simulink model "fu_simu_png_radome_origin"  (R2020a)
settings: Solver=ode4  StartTime=0.0  StopTime=20  FixedStep=0.001  RelTol=1e-3
values from neighbouring files (symbols this model uses):
  N = 4    [initial.m]
  T_alpha = 1    [initial.m]
  tau = 0.1    [initial.m]
  V_M = 500    [initial.m]
libraries: simulink x1
settings Model: Creator=admin  LastModifiedBy=anwaei

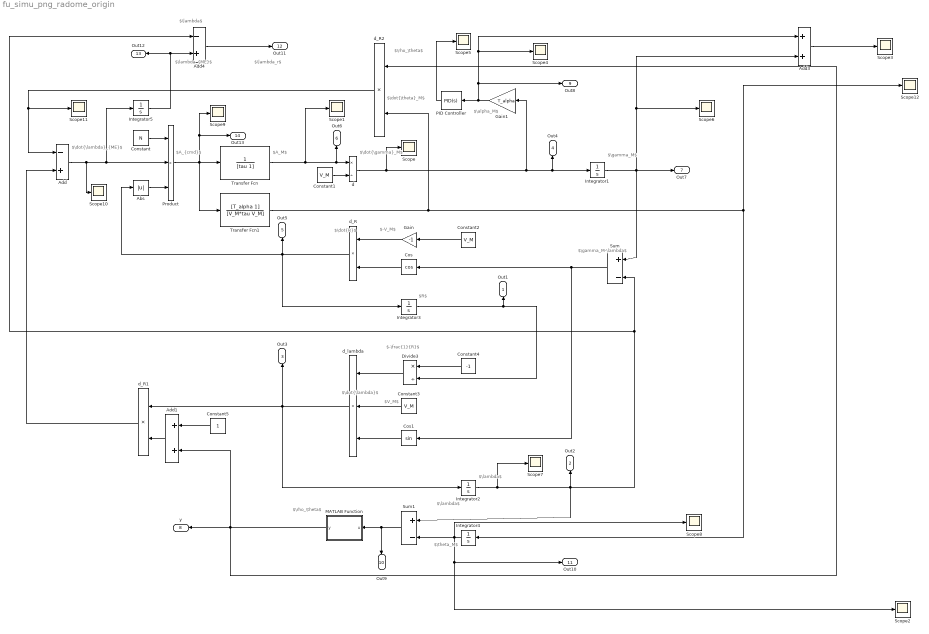
== system fu_simu_png_radome_origin ==
  note: $\dot{\lambda}$
  note: $\lambda$
  note: $\gamma_M$
  note: $-\frac{1}{R}$
  note: $V_M$
  note: $\gamma_M-\lambda$
  note: $-V_M$
  note: $\dot{R}$
  note: $A_{cmd}$
  note: $A_M$
  note: $\dot{\gamma}_M$
  note: $R$
  note: $\dot{\theta}_M$
  note: $\dot{\lambda}_{ME}$
  note: $\theta_M$
  note: $\lambda$
  note: $\rho_\theta$
  note: $\rho_\theta$
  note: $\alpha_M$
  note: $\lambda_{ME}$
  note: $\lambda$
  note: $\lambda_r$
  Abs : Abs
  Add : Sum  Inputs=-+
  Add1 : Sum
  Add3 : Sum
  Add4 : Sum  Inputs=-+
  Constant : Constant  Value=N
  Constant1 : Constant  Value=V_M
  Constant2 : Constant  Value=V_M
  Constant3 : Constant  Value=V_M
  Constant4 : Constant  Value=-1
  Constant5 : Constant
  Cos : Trigonometry  Operator=cos
  Cos1 : Trigonometry
  Divide3 : Product  Inputs=*/
  Gain : Gain  Gain=-1
  Gain1 : Gain  Gain=T_alpha
  Integrator1 : Integrator
  Integrator2 : Integrator  InitialCondition=0.0997
  Integrator3 : Integrator  InitialCondition=10050
  Integrator4 : Integrator
  Integrator5 : Integrator  InitialCondition=0.1021925
  MATLAB Function : MATLAB Function  TreatAsAtomicUnit=on
  PID Controller : simulink/Continuous/PID Controller  Controller=PID  Form=Parallel  TimeDomain=Continuous-time  UseExternalTs=off  SampleTime=-1  IntegratorMethod=Forward Euler  FilterMethod=Forward Euler  ControllerParametersSource=internal  P=0  I=0  D=1  UseFilter=on  N=1000  TunerSelectOption=Transfer Function Based (PID Tuner App)  InitialConditionSource=internal  InitialConditionForIntegrator=0  InitialConditionForFilter=0  DifferentiatorICPrevScaledInput=0  ExternalReset=none  TrackingMode=off  Kt=1  LimitOutput=off  UpperSaturationLimit=inf  LowerSaturationLimit=-inf  LinearizeAsGain=on  AntiWindupMode=none  Kb=1  POutMin=[]  POutMax=[]  IOutMin=[]  IOutMax=[]  DOutMin=[]  DOutMax=[]  NOutMin=[]  NOutMax=[]  SumOutMin=[]  SumOutMax=[]  SaturationOutMin=[]  SaturationOutMax=[]  PParamMin=[]  PParamMax=[]  IParamMin=[]  IParamMax=[]  DParamMin=[]  DParamMax=[]  NParamMin=[]  NParamMax=[]  KbParamMin=[]  KbParamMax=[]  KtParamMin=[]  KtParamMax=[]  KbOutMin=[]  KbOutMax=[]  KtOutMin=[]  KtOutMax=[]  IntegratorOutMin=[]  IntegratorOutMax=[]  FilterOutMin=[]  FilterOutMax=[]  SumI1OutMin=[]  SumI1OutMax=[]  SumI2OutMin=[]  SumI2OutMax=[]  SumI3OutMin=[]  SumI3OutMax=[]  SumI4OutMin=[]  SumI4OutMax=[]  SumDOutMin=[]  SumDOutMax=[]  DifferentiatorOutMin=[]  DifferentiatorOutMax=[]  FilterDiffOutCoefMin=[]  FilterDiffOutCoefMax=[]  ReciprocalOutMin=[]  ReciprocalOutMax=[]  SumDenOutMin=[]  SumDenOutMax=[]  SumNumOutMin=[]  SumNumOutMax=[]  DivideOutMin=[]  DivideOutMax=[]  UdiffTsProdOutMin=[]  UdiffTsProdOutMax=[]  NTsProdOutMin=[]  NTsProdOutMax=[]  UintegralTsProdOutMin=[]  UintegralTsProdOutMax=[]  UngainTsProdOutMin=[]  UngainTsProdOutMax=[]  IntegratorContinuousStateAttributes=''  IntegratorStateMustResolveToSignalObject=off  IntegratorRTWStateStorageClass=Auto  FilterContinuousStateAttributes=''  FilterStateMustResolveToSignalObject=off  FilterRTWStateStorageClass=Auto  ParallelPVariant=InternalParameters  IdealPVariant=Disabled  IVariant=InternalParameters  DVariant=InternalParameters  IntegratorVariant=Continuous  SatVariant=Disabled  AWVariant=Passthrough  PCopyVariant=Disabled  TRVariant=Disabled  FdbkBlocksVariant=Forward  IdealPFdbkVariant=Disabled  SatFdbkVariant=Disabled  DerivativeFilterVariant=ContFilter  NVariant=InternalParameters  NCopyVariant=Disabled  FilterICVariant=InternalICsFilter  IntegratorICVariant=InternalICs  ExternalResetVariant=Disabled  TRSumVariant=Passthrough  SumFdbkVariant=Disabled  SumVariant=Sum_PID  TsampFilterVariant=InternalTs  TsampNgainVariant=Passthrough  TsampIntegralVariant=Passthrough
  Product : Product  Inputs=3
  Scope{,1..12} (13 alike) : Scope
  Sum : Sum  Inputs=+|-
  Sum1 : Sum  Inputs=+|-
  Transfer Fcn : TransferFcn  Denominator=[tau 1]
  Transfer Fcn1 : TransferFcn  Numerator=[T_alpha 1]  Denominator=[V_M*tau V_M]
  d : Product  Inputs=*/
  d_R : Product  Inputs=**
  d_R1 : Product  Inputs=**
  d_R2 : Product  Inputs=**
  d_lambda : Product  Inputs=***
  Out1 : Outport
  Out2 : Outport  Port=2
  Out3 : Outport  Port=3
  Out4 : Outport  Port=4
  Out5 : Outport  Port=5
  Out6 : Outport  Port=6
  Out7 : Outport  Port=7
  y : Outport  Port=8
  Out8 : Outport  Port=9
  Out9 : Outport  Port=10
  Out10 : Outport  Port=11
  Out11 : Outport  Port=12
  Out12 : Outport  Port=13
  Out13 : Outport  Port=14
  wires:
  Transfer Fcn/1 -> Scope1/1, d/1, Out6/1
  Integrator3/1 -> Out1/1, Divide3/2
  Constant/1 -> Product/1
  Product/1 -> Transfer Fcn1/1, Out13/1, Scope9/1, Transfer Fcn/1
  Abs/1 -> Product/3
  Constant1/1 -> d/2
  Gain/1 -> d_R/1
  Constant2/1 -> Gain/1
  Cos/1 -> d_R/2
  d_R/1 -> Out5/1, Integrator3/1, Abs/1
  Divide3/1 -> d_lambda/1
  Constant3/1 -> d_lambda/2
  Cos1/1 -> d_lambda/3
  Sum/1 -> Cos1/1, Cos/1
  Integrator1/1 -> Scope6/1, Add3/2, Out7/1, Sum/1
  d_lambda/1 -> Integrator2/1, d_R1/1, Out3/1
  Constant4/1 -> Divide3/1
  d/1 -> Scope/1, Gain1/1, Out4/1, Integrator1/1
  Add/1 -> Scope10/1, Product/2, Integrator5/1
  Add1/1 -> d_R1/2
  Constant5/1 -> Add1/1
  d_R1/1 -> Add/2
  PID Controller/1 -> Scope5/1
  Transfer Fcn1/1 -> d_R2/2, Scope12/1, Integrator4/1
  d_R2/1 -> Scope11/1, Add/1
  Integrator4/1 -> Scope8/1, Out10/1, Scope2/1, Sum1/2
  Sum1/1 -> Out9/1, MATLAB Function/1(u)
  MATLAB Function/1(y) -> y/1, Add1/2, d_R2/1
  Gain1/1 -> PID Controller/1, Add3/1, Scope4/1, Out8/1
  Add3/1 -> Scope3/1
  Integrator5/1 -> Add4/2, Out12/1
  Integrator2/1 -> Scope7/1, Sum1/1, Add4/1, Sum/2, Out2/1
  Add4/1 -> Out11/1

== matlab function fu_simu_png_radome_origin/MATLAB Function ==
  data: u input; y output
function y = fcn(u)

%%
r=-0.5;
zeta=4;
p=1;

if u<0
    a=exp(zeta*u);
    b=zeta*sin(2*pi*u/p);
    c=2*pi/p*cos(2*pi*u/p);
else
    a=exp(-zeta*u);
    b=-zeta*sin(2*pi*u/p);
    c=2*pi/p*cos(2*pi*u/p);
end

y=r*a*(b+c);
y=y/rad2deg(1);

%%
% y=0.025;
% y=0.05;
% y=-0.025;
